simulink model "feedback_yd"  (R2022b)
settings: Solver=FixedStepAuto  StartTime=0.0  StopTime=15  FixedStep=0.001  RelTol=1e-3
model workspace (MAT data in the model file):
  k1 = Simulink.Parameter
  k1.Value = 1000
  k1.DataType = 'auto'
  k1.Complexity = 'real'
  k1.Dimensions = [1 1]
  k2 = Simulink.Parameter
  k2.Value = 100
  k2.DataType = 'auto'
  k2.Complexity = 'real'
  k2.Dimensions = [1 1]
values from neighbouring files (symbols this model uses):
  k_p1 = 30    [gains.m]
  k_p2 = 30    [gains.m]
undefined symbols (not defined in the file or in its folder): obstacle_x, obstacle_y, overtake_data, overtake_time, x_start, y_start
libraries: robotmobilelib x4, dspsigops x2
settings Model: Creator=thoma  LastModifiedBy=borgh

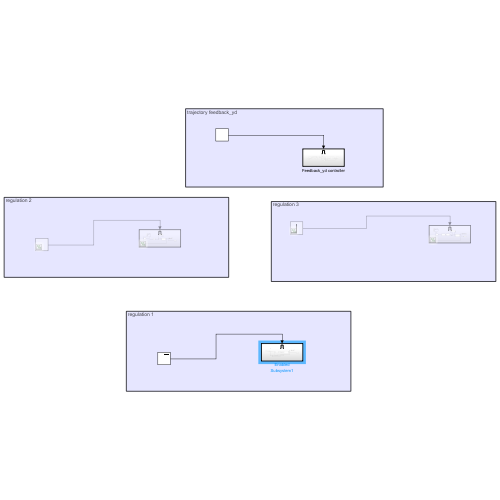
[thumbnail: Simulink's stored preview of the top-level diagram]
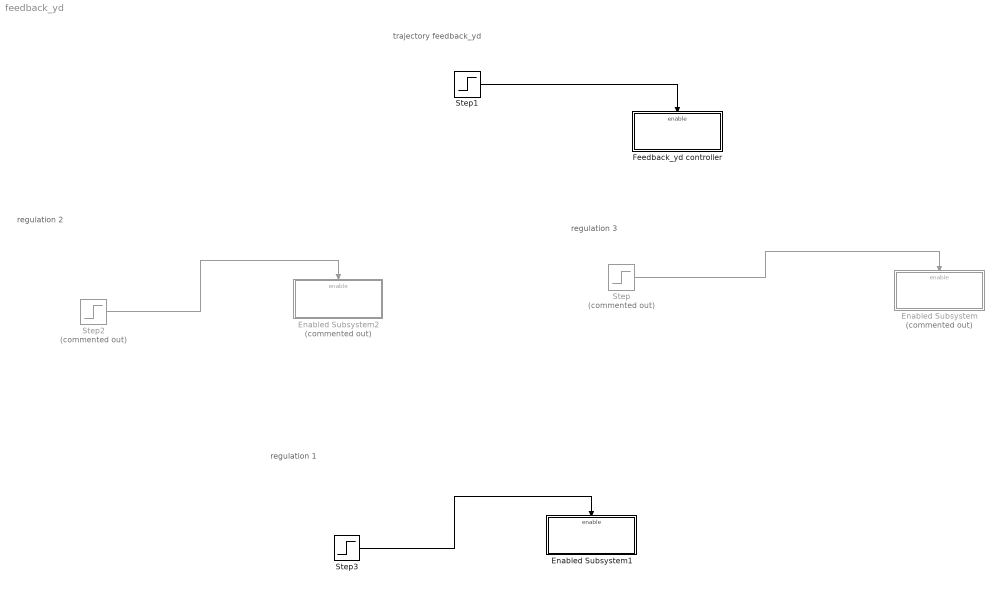
== system feedback_yd ==
  note: regulation 3
  note: trajectory feedback_yd
  note: regulation 2
  note: regulation 1
  Enabled Subsystem : Subsystem  Commented=on  TreatAsAtomicUnit=on
  Enabled Subsystem1 : Subsystem  TreatAsAtomicUnit=on
  Enabled Subsystem2 : Subsystem  Commented=on  TreatAsAtomicUnit=on
  Feedback_yd controller : Subsystem  TreatAsAtomicUnit=on
  Step : Step  Commented=on  Time=10  SampleTime=0
  Step1 : Step  Time=10  Before=1  After=0  SampleTime=0
  Step2 : Step  Commented=on  Time=10  SampleTime=0
  Step3 : Step  Time=10  SampleTime=0
  wires:
  Step2/1 -> Enabled Subsystem2/Enable
  Step1/1 -> Feedback_yd controller/Enable
  Step/1 -> Enabled Subsystem/Enable
  Step3/1 -> Enabled Subsystem1/Enable

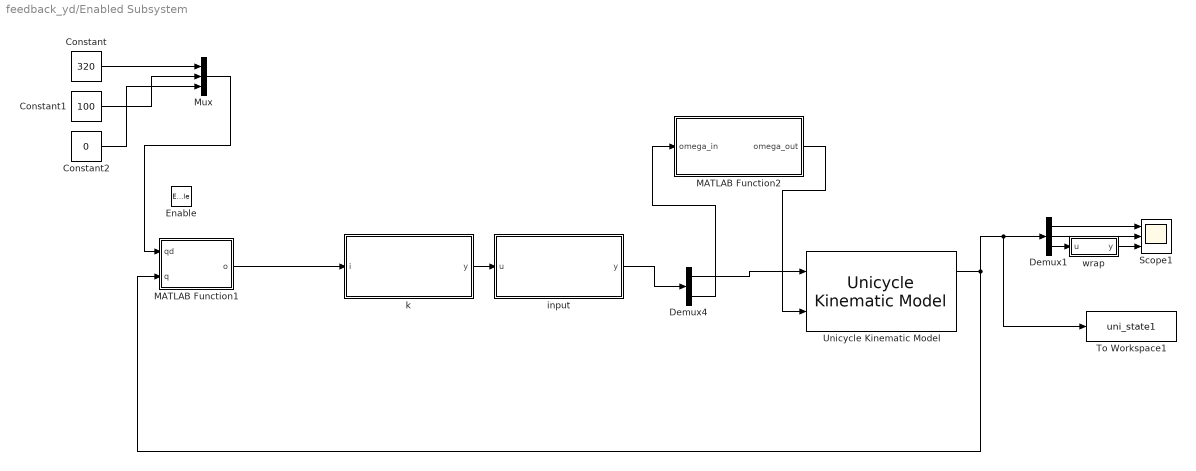
== system feedback_yd/Enabled Subsystem ==
  Enable : EnablePort
  Constant : Constant  Value=320
  Constant1 : Constant  Value=100
  Constant2 : Constant  Value=0
  Demux1 : Demux  Outputs=3
  Demux4 : Demux  Outputs=2
  MATLAB Function1 : MATLAB Function  TreatAsAtomicUnit=on
  MATLAB Function2 : MATLAB Function  TreatAsAtomicUnit=on
  Mux : Mux  Inputs=3
  Scope1 : Scope  NumInputPorts=3
  To Workspace1 : ToWorkspace  VariableName=uni_state1  SaveFormat=Structure With Time  SampleTime=0.001
  Unicycle Kinematic Model : robotmobilelib/Unicycle Kinematic Model  VehicleInputs=Vehicle Speed & Heading Angular Velocity  WheelRadius=2  WheelSpeedRange=[-Inf Inf]  InitialState=[125,60,0]  SimulateUsing=Interpreted execution
  input : MATLAB Function  TreatAsAtomicUnit=on
  k : MATLAB Function  TreatAsAtomicUnit=on
  wrap : MATLAB Function  TreatAsAtomicUnit=on
  wires:
  Constant/1 -> Mux/1
  Constant1/1 -> Mux/2
  Constant2/1 -> Mux/3
  Demux1/2 -> Scope1/2
  wrap/1(y) -> Scope1/3
  Unicycle Kinematic Model/1 -> To Workspace1/1, Demux1/1, MATLAB Function1/2(q)
  input/1(y) -> Demux4/1
  Demux1/3 -> wrap/1(u)
  k/1(y) -> input/1(u)
  Demux1/1 -> Scope1/1
  MATLAB Function1/1(o) -> k/1(i)
  Demux4/1 -> Unicycle Kinematic Model/1
  Mux/1 -> MATLAB Function1/1(qd)
  Demux4/2 -> MATLAB Function2/1(omega_in)
  MATLAB Function2/1(omega_out) -> Unicycle Kinematic Model/2

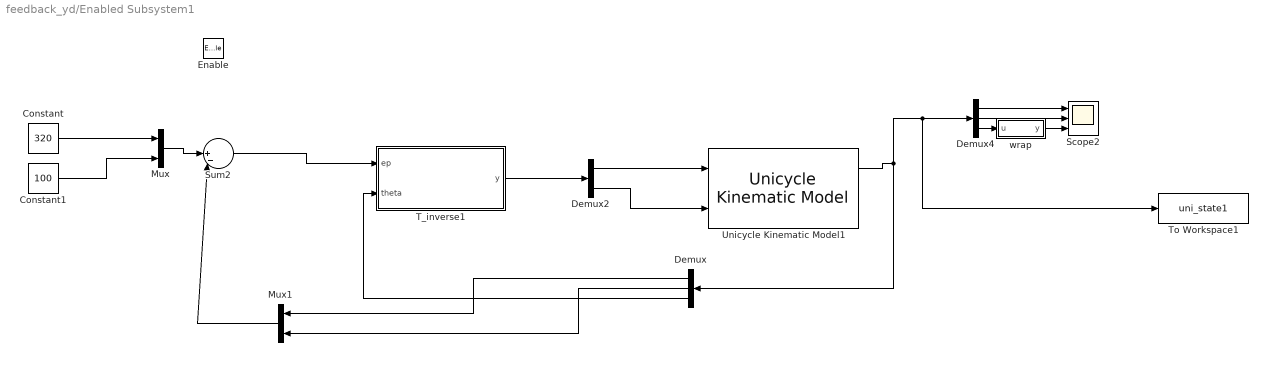
== system feedback_yd/Enabled Subsystem1 ==
  Enable : EnablePort
  Constant : Constant  Value=320
  Constant1 : Constant  Value=100
  Demux : Demux  Outputs=3
  Demux2 : Demux  Outputs=2
  Demux4 : Demux  Outputs=3
  Mux : Mux  Inputs=2
  Mux1 : Mux  Inputs=2
  Scope2 : Scope  NumInputPorts=3
  Sum2 : Sum  Inputs=||+-|
  T_inverse1 : MATLAB Function  TreatAsAtomicUnit=on
  To Workspace1 : ToWorkspace  VariableName=uni_state1  SaveFormat=Structure With Time  SampleTime=0.001
  Unicycle Kinematic Model1 : robotmobilelib/Unicycle Kinematic Model  VehicleInputs=Vehicle Speed & Heading Angular Velocity  WheelRadius=2  WheelSpeedRange=[-Inf Inf]  InitialState=[125,60,0]  SimulateUsing=Interpreted execution
  wrap : MATLAB Function  TreatAsAtomicUnit=on
  wires:
  wrap/1(y) -> Scope2/3
  Demux4/1 -> Scope2/1
  Demux4/2 -> Scope2/2
  Demux4/3 -> wrap/1(u)
  Sum2/1 -> T_inverse1/1(ep)
  Demux/1 -> Mux1/1
  Demux2/2 -> Unicycle Kinematic Model1/2
  Mux1/1 -> Sum2/2
  Demux2/1 -> Unicycle Kinematic Model1/1
  Unicycle Kinematic Model1/1 -> To Workspace1/1, Demux4/1, Demux/1
  T_inverse1/1(y) -> Demux2/1
  Demux/2 -> Mux1/2
  Demux/3 -> T_inverse1/2(theta)
  Constant1/1 -> Mux/2
  Constant/1 -> Mux/1
  Mux/1 -> Sum2/1

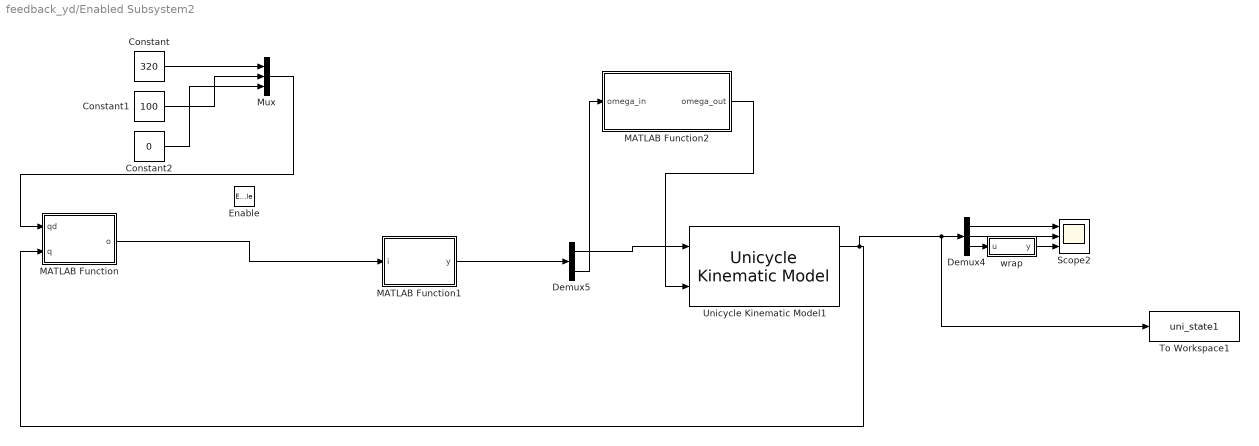
== system feedback_yd/Enabled Subsystem2 ==
  Enable : EnablePort
  Constant : Constant  Value=320
  Constant1 : Constant  Value=100
  Constant2 : Constant  Value=0
  Demux4 : Demux  Outputs=3
  Demux5 : Demux  Outputs=2
  MATLAB Function : MATLAB Function  TreatAsAtomicUnit=on
  MATLAB Function1 : MATLAB Function  TreatAsAtomicUnit=on
  MATLAB Function2 : MATLAB Function  TreatAsAtomicUnit=on
  Mux : Mux  Inputs=3
  Scope2 : Scope  NumInputPorts=3
  To Workspace1 : ToWorkspace  VariableName=uni_state1  SaveFormat=Structure With Time  SampleTime=0.001
  Unicycle Kinematic Model1 : robotmobilelib/Unicycle Kinematic Model  VehicleInputs=Vehicle Speed & Heading Angular Velocity  WheelRadius=2  WheelSpeedRange=[-Inf Inf]  InitialState=[125,60,0]  SimulateUsing=Interpreted execution
  wrap : MATLAB Function  TreatAsAtomicUnit=on
  wires:
  Demux5/1 -> Unicycle Kinematic Model1/1
  wrap/1(y) -> Scope2/3
  MATLAB Function/1(o) -> MATLAB Function1/1(i)
  MATLAB Function1/1(y) -> Demux5/1
  Demux4/1 -> Scope2/1
  Demux4/2 -> Scope2/2
  Demux4/3 -> wrap/1(u)
  Unicycle Kinematic Model1/1 -> To Workspace1/1, Demux4/1, MATLAB Function/2(q)
  Constant/1 -> Mux/1
  Constant1/1 -> Mux/2
  Constant2/1 -> Mux/3
  Mux/1 -> MATLAB Function/1(qd)
  Demux5/2 -> MATLAB Function2/1(omega_in)
  MATLAB Function2/1(omega_out) -> Unicycle Kinematic Model1/2

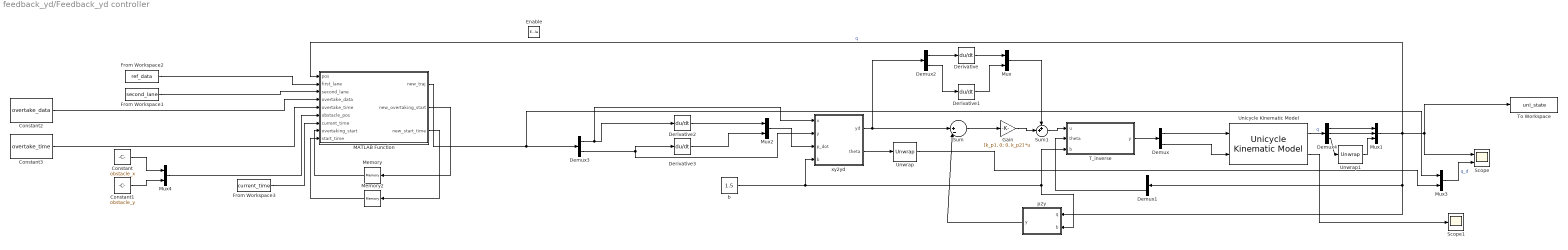
== system feedback_yd/Feedback_yd controller ==
  Enable : EnablePort
  Constant : Constant  Value=obstacle_x
  Constant1 : Constant  Value=obstacle_y
  Constant2 : Constant  Value=overtake_data
  Constant3 : Constant  Value=overtake_time
  Demux : Demux  Outputs=2
  Demux1 : Demux  Outputs=3
  Demux2 : Demux  Outputs=2
  Demux3 : Demux  Outputs=2
  Demux4 : Demux  Outputs=3
  Derivative{,1..3} (4 alike) : Derivative
  From Workspace1 : FromWorkspace  VariableName=second_lane
  From Workspace2 : FromWorkspace  VariableName=ref_data
  From Workspace3 : FromWorkspace  VariableName=current_time
  Gain : Gain  Gain=[k_p1, 0; 0, k_p2]  Multiplication=Matrix(K*u)
  MATLAB Function : MATLAB Function  TreatAsAtomicUnit=on
  Memory : Memory
  Memory2 : Memory
  Mux{,2..4} (4 alike) : Mux  Inputs=2
  Mux1 : Mux  Inputs=3
  Scope : Scope  NumInputPorts=2
  Scope1 : Scope
  Sum : Sum  Inputs=||+-|
  Sum1 : Sum  Inputs=++|
  T_inverse : MATLAB Function  TreatAsAtomicUnit=on
  To Workspace : ToWorkspace  VariableName=uni_state  SaveFormat=Structure With Time  SampleTime=0.01
  Unicycle Kinematic Model : robotmobilelib/Unicycle Kinematic Model  VehicleInputs=Vehicle Speed & Heading Angular Velocity  WheelRadius=2  WheelSpeedRange=[-Inf Inf]  InitialState=[x_start; y_start; 0]  SimulateUsing=Interpreted execution
  Unwrap : dspsigops/Unwrap  tol=pi  InputProcessing=Columns as channels (frame based)  running=off
  Unwrap1 : dspsigops/Unwrap  tol=pi  InputProcessing=Columns as channels (frame based)  running=off
  b : Constant  Value=1.5
  p2y : MATLAB Function  TreatAsAtomicUnit=on
  xy2yd : MATLAB Function  TreatAsAtomicUnit=on
  wires:
  Mux2/1 -> xy2yd/3(p_dot)
  Derivative3/1 -> Mux2/2
  Gain/1 -> Sum1/2
  T_inverse/1(y) -> Demux/1
  Demux3/1 -> xy2yd/1(x), Derivative2/1
  Demux3/2 -> Derivative3/1, xy2yd/2(y)
  Mux1/1 -> p2y/1(q), Demux1/1, MATLAB Function/1(pos), Scope/1, To Workspace/1  "q"
  p2y/1(y) -> Sum/2
  Demux/2 -> Unicycle Kinematic Model/2
  xy2yd/1(yd) -> Demux2/1, Sum/1
  Derivative2/1 -> Mux2/1
  Demux2/2 -> Derivative1/1
  Derivative/1 -> Mux/1
  Derivative1/1 -> Mux/2
  Mux/1 -> Sum1/1
  Sum/1 -> Gain/1
  Demux2/1 -> Derivative/1
  xy2yd/2(theta) -> Unwrap/1
  Demux1/3 -> T_inverse/2(theta)
  Mux3/1 -> Scope/2  "q_d"
  Sum1/1 -> T_inverse/1(u)
  Demux/1 -> Unicycle Kinematic Model/1
  b/1 -> xy2yd/4(b), T_inverse/3(b), p2y/2(b)
  From Workspace1/1 -> MATLAB Function/3(second_lane)
  From Workspace2/1 -> MATLAB Function/2(first_lane)
  MATLAB Function/1(new_traj) -> Mux3/1, Demux3/1
  Mux4/1 -> MATLAB Function/6(obstacle_pos)
  Constant1/1 -> Mux4/2
  Constant/1 -> Mux4/1
  From Workspace3/1 -> MATLAB Function/7(current_time)
  Memory/1 -> MATLAB Function/8(overtaking_start)
  MATLAB Function/2(new_overtaking_start) -> Memory/1
  MATLAB Function/3(new_start_time) -> Memory2/1
  Memory2/1 -> MATLAB Function/9(start_time)
  Constant2/1 -> MATLAB Function/4(overtake_data)
  Constant3/1 -> MATLAB Function/5(overtake_time)
  Unwrap/1 -> Mux3/2
  Unwrap1/1 -> Mux1/3
  Demux4/1 -> Mux1/1
  Unicycle Kinematic Model/1 -> Demux4/1  "q"
  Demux4/2 -> Mux1/2
  Demux4/3 -> Unwrap1/1
  Unicycle Kinematic Model/2 -> Scope1/1

== matlab function feedback_yd/Enabled Subsystem2/MATLAB Function2 ==
  data: omega_in input; omega_out output
function omega_out = check_omega(omega_in)
    % Check if omega (angular velocity) is finite
    if ~isfinite(omega_in)
        omega_out = 0;  % Set omega to a default value, e.g., 0 if it is NaN or Inf
    else
        omega_out = omega_in;  % Otherwise, pass the input value
    end
end

== matlab function feedback_yd/Enabled Subsystem2/wrap ==
  data: u input; y output
function y = fcn(u)

y =mod(u+pi,2*pi)-pi;

== matlab function feedback_yd/Enabled Subsystem/k ==
  data: i input; y output
function y = fcn(i)
k1=20;
k2=100;
k3=20;
rho=i(1);
gamma=i(2);
delta=i(3);
u=k1*cos(gamma);
w=k2*gamma+(k1* ((sin(gamma)*cos(gamma))/gamma) * (gamma+k3*delta));
y = [rho;u;w];

== matlab function feedback_yd/Enabled Subsystem/wrap ==
  data: u input; y output
function y = fcn(u)

y =mod(u+pi,2*pi)-pi;

== matlab function feedback_yd/Enabled Subsystem1/wrap ==
  data: u input; y output
function y = fcn(u)

y =mod(u+pi,2*pi)-pi;

== matlab function feedback_yd/Enabled Subsystem1/T_inverse1 ==
  data: ep input; y output; theta input
function y = fcn(ep,theta)
theta=mod(theta+pi,2*pi)-pi;
kv=40;
kw=50;
v=kv*(ep(1)*cos(theta)+ep(2)*sin(theta));
w=kw*(atan2(-ep(2),-ep(1))+pi-theta);
y = [v;w];

== matlab function feedback_yd/Feedback_yd controller/p2y ==
  data: q input; y output; b input
function y = fcn(q,b)
x=q(1);
yi=q(2);
theta=q(3);
y1=x+b*cos(theta);
y2=yi+b*sin(theta);
y=[y1;y2];

== matlab function feedback_yd/Feedback_yd controller/T_inverse ==
  data: u input; y output; theta input; b input
function y = fcn(u,theta,b)
T_inverse=[cos(theta),sin(theta);-sin(theta)/b,cos(theta)/b];
vet=T_inverse*u;
a=vet(1);
w=vet(2);
y = vet;

== matlab function feedback_yd/Feedback_yd controller/xy2yd ==
  data: x input; y input; p_dot input; yd output; b input; theta output
function [yd, theta] = fcn(x,y, p_dot,b)
v_x = p_dot(1);
if abs(v_x) <= 1e-4
    v_x = sign(v_x)*1e-4;
end
v_y = p_dot(2);
theta = atan2(v_y, v_x);
y1=x+b*cos(theta);
y2=y+b*sin(theta);
yd=[y1;y2];

== matlab function feedback_yd/Enabled Subsystem/MATLAB Function2 ==
  data: omega_in input; omega_out output
function omega_out = check_omega(omega_in)
    % Check if omega (angular velocity) is finite
    if ~isfinite(omega_in)
        omega_out = 0;  % Set omega to a default value, e.g., 0 if it is NaN or Inf
    else
        omega_out = omega_in;  % Otherwise, pass the input value
    end
end

== matlab function feedback_yd/Feedback_yd controller/MATLAB Function ==
  data: pos input; first_lane input; new_traj output; second_lane input; overtake_data input; overtake_time input; obstacle_pos input size=[2]; current_time input; overtaking_start input; new_overtaking_start output; new_start_time output; start_time input
function [new_traj, new_overtaking_start, new_start_time]  = fcn(pos,first_lane, second_lane, overtake_data, overtake_time, obstacle_pos, current_time, overtaking_start, start_time)
detection_margin_x = 85; % Detection range in x-direction
detection_margin_y = 55; % Detection range in y-direction
early_detection_distance = 60; % Distance ahead of obstacle to start overtaking
% Check if obstacle is within detection range and ahead of the obstacle   
if ~overtaking_start   
    if (abs(pos(1) - obstacle_pos(1)) < detection_margin_x && abs(pos(2) - obstacle_pos(2)) < detection_margin_y) && pos(1) < obstacle_pos(1) + early_detection_distance
        new_overtaking_start = 1;
        new_start_time = current_time;
    else
        new_overtaking_start = overtaking_start;
        new_start_time = start_time;
    end
    idx = 1;
else
    idx = find(abs(overtake_time - (current_time - start_time)) <= 1e-3, 1);
    if ~isempty(idx)
        new_overtaking_start = overtaking_start;
    else
        new_overtaking_start = 0;
        idx = 1;
    end
    new_start_time = start_time;
end
new_traj = first_lane + (second_lane-first_lane)*overtake_data(idx);

== matlab function feedback_yd/Enabled Subsystem/MATLAB Function1 ==
  data: qd input; o output; q input
function o = fcn(qd,q)
xi=q(1);
yi=q(2);
thetai=q(3);
x=-(qd(1)-xi);
y=-(qd(2)-yi);
theta=-(qd(3)-thetai);
theta=mod(theta+pi,2*pi)-pi;
rho=sqrt(x^2+y^2);
gamma=atan2(y,x)+pi-theta;
delta=gamma+theta;
delta=mod(delta+pi,2*pi)-pi;
gamma=mod(gamma+pi,2*pi)-pi;
o = [rho;gamma;delta];

== matlab function feedback_yd/Enabled Subsystem/input ==
  data: u input; y output
function y = fcn(u)
v=u(2)*u(1);
w=u(3);
y = [v;w];

== matlab function feedback_yd/Enabled Subsystem2/MATLAB Function ==
  data: qd input; o output; q input
function o = fcn(qd,q)
xi=q(1);
yi=q(2);
thetai=q(3);
x=-(qd(1)-xi);
y=-(qd(2)-yi);
theta=-(qd(3)-thetai);
rho=sqrt(x^2+y^2);
gamma=atan2(y,x)+pi-theta;
delta=gamma+theta;
delta=mod(delta+pi,2*pi)-pi;
gamma=mod(gamma+pi,2*pi)-pi;
o = [rho;gamma;delta];

== matlab function feedback_yd/Enabled Subsystem2/MATLAB Function1 ==
  data: i input; y output
function y = fcn(i)
k1=20;
k2=30;
k3=4;
rho=i(1);
gamma=i(2);
delta=i(3);
v=k1*rho*cos(gamma);
w=k2*gamma+(k1* ((sin(gamma)*cos(gamma))/gamma) * (gamma+k3*delta));
y = [v;w];
